simulink library "digtwin_labo_lib"  (R2025b)
settings: Solver=VariableStepAuto  StartTime=0.0  StopTime=10.0  RelTol=1e-3
undefined symbols (not defined in the file): b1_num, b2_num, COUNTS_PER_TURN, COUNTS_PER_TURN_MOT, COUNTS_PER_TURN_PEND, dspblkCoreblockFVToolHelper, g_num, gcbh, l_num, m_num, MOTOR_VEL_RESOLUTION_DIV, Nv2filt, PEND_VEL_RESOLUTION_DIV, q1_0, q2_0, r_num, satlimits, STEPS_PER_TURN, T01_num0, T12_num0, T_SAMPLE, v1_0, v2_0, X, Y, Z
libraries: sm_lib x24, nesl_utility x14, fl_lib x4, ee_lib x4, $bdroot x4, simulink x2, raspberrypiCommlib x2
(part 2 of 2)

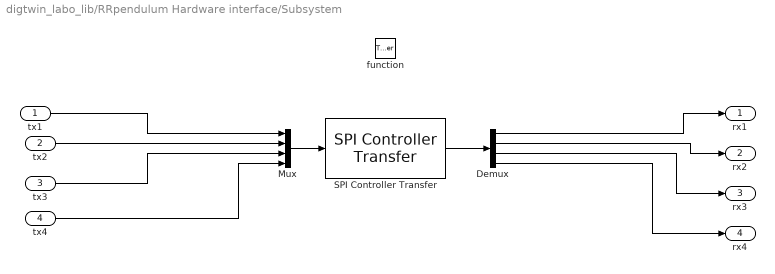
== system digtwin_labo_lib/RRpendulum Hardware interface/Subsystem ==
  tx1 : Inport
  tx2 : Inport  Port=2
  tx3 : Inport  Port=3
  tx4 : Inport  Port=4
  function : TriggerPort  TriggerType=function-call  VariantControl=(inherit)
  Demux : Demux
  Mux : Mux
  SPI Controller Transfer : raspberrypiCommlib/SPI Controller Transfer  BoardProperty=Pi 4 Model B  SSPin=SPI0_CE0  SPIModule=uint32(0)  Mode=Master  BusSpeed=1000000  Pin=uint32(0)  FirstBitToTransfer=Most significant bit (MSB)  ClockMode=0  BlockFunction=Transfer  RegisterAddress=0  OutputDataType=int8  OutputDataLength=1
  rx1 : Outport
  rx2 : Outport  Port=2
  rx3 : Outport  Port=3
  rx4 : Outport  Port=4
  wires:
  Demux/4 -> rx4/1
  tx4/1 -> Mux/4
  Demux/3 -> rx3/1
  tx3/1 -> Mux/3
  Demux/2 -> rx2/1
  Mux/1 -> SPI Controller Transfer/1
  tx2/1 -> Mux/2
  Demux/1 -> rx1/1
  tx1/1 -> Mux/1
  SPI Controller Transfer/1 -> Demux/1
